simulink model "aufgabe1_linear_reibung_c10_anfangsbedingung2"  (R2023b)
settings: Solver=FixedStepAuto  StartTime=0.0  StopTime=10.0  FixedStep=0.001  RelTol=1e-3
settings Model: Creator=serkan  LastModifiedBy=serkan

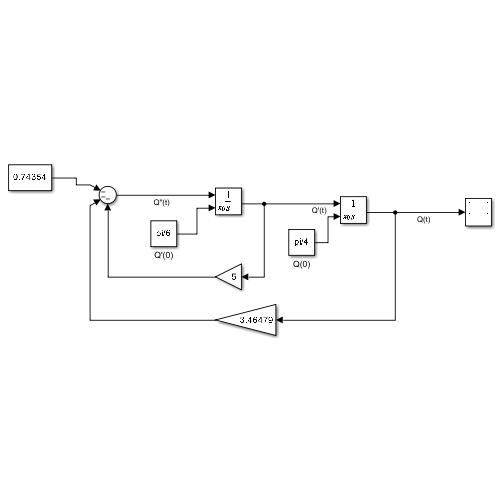
[thumbnail: Simulink's stored preview of the top-level diagram]
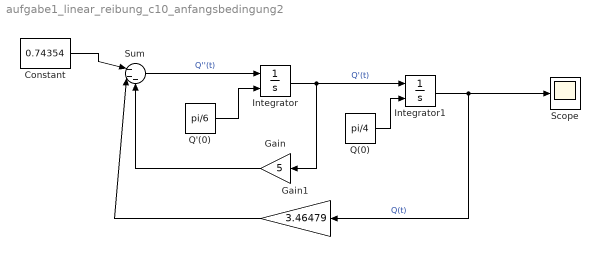
== system aufgabe1_linear_reibung_c10_anfangsbedingung2 ==
  Constant : Constant  Value=0.74354
  Gain : Gain  Gain=5
  Gain1 : Gain  Gain=3.46479
  Integrator : Integrator  InitialConditionSource=external
  Integrator1 : Integrator  InitialConditionSource=external
  Q'(0) : Constant  Value=pi/6
  Q(0) : Constant  Value=pi/4
  Scope : Scope
  Sum : Sum  Inputs=|---
  wires:
  Integrator/1 -> Integrator1/1, Gain/1  "Q'(t)"
  Integrator1/1 -> Scope/1, Gain1/1  "Q(t)"
  Q'(0)/1 -> Integrator/2
  Gain/1 -> Sum/3
  Sum/1 -> Integrator/1  "Q''(t)"
  Constant/1 -> Sum/1
  Gain1/1 -> Sum/2
  Q(0)/1 -> Integrator1/2
